simulink model "funevent"  (R2023a)
settings: Solver=FixedStepDiscrete  StartTime=0.0  StopTime=10.0  FixedStep=1e-3  RelTol=1e-3
settings Model: Creator=Egypt_Laptop  LastModifiedBy=Egypt_Laptop

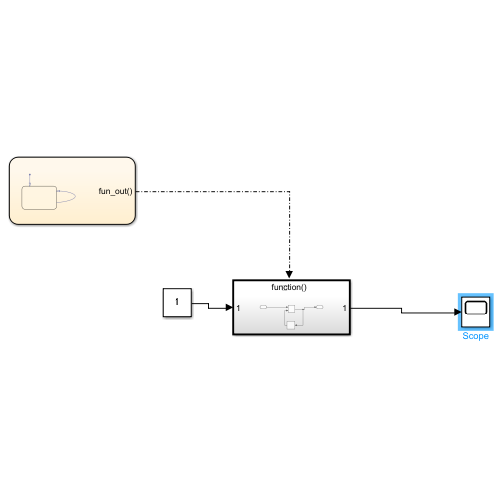
[thumbnail: Simulink's stored preview of the top-level diagram]
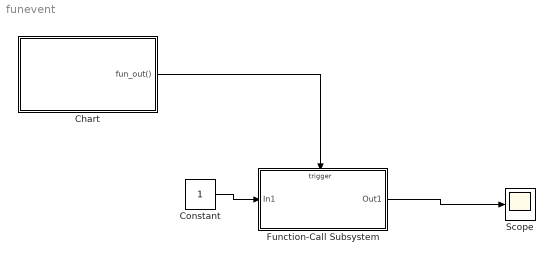
== system funevent ==
  Chart : Stateflow chart  TreatAsAtomicUnit=on
  Constant : Constant
  Function-Call Subsystem : Subsystem  TreatAsAtomicUnit=on
  Scope : Scope
  wires:
  Constant/1 -> Function-Call Subsystem/1(In1)
  Function-Call Subsystem/1(Out1) -> Scope/1
  Chart/1(fun_out()) -> Function-Call Subsystem/Trigger

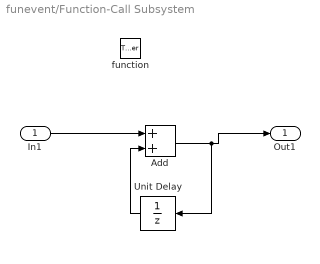
== system funevent/Function-Call Subsystem ==
  In1 : Inport
  function : TriggerPort  TriggerType=function-call  VariantControl=(inherit)
  Add : Sum
  Unit Delay : UnitDelay  SampleTime=-1  HasFrameUpgradeWarning=on
  Out1 : Outport
  wires:
  Add/1 -> Unit Delay/1, Out1/1
  In1/1 -> Add/1
  Unit Delay/1 -> Add/2

== stateflow chart funevent/Chart ==
  state S1
  (default) -> S1
  S1 -> S1 : after(1,sec){fun_out}
  events: fun_out local FUNCTION_CALL_EVENT; fun_out output FUNCTION_CALL_EVENT
